simulink model "oloop2"  (Simulink 3.00)
settings: Solver=ode45  SolverMode=SingleTasking  StartTime=0.0  StopTime=60  MaxStep=1  RelTol=1e-7  AbsTol=1e-7
undefined symbols (not defined in the file): sfunyst, uaero0, uprop0
libraries: fbuttons x5, fdclib10 x1, wndlib2 x1
settings Model: SaveTime=off  SaveOutput=off  RTWTemplateMakefile=grt_vc.tmf  LastModifiedBy=Dutchroll

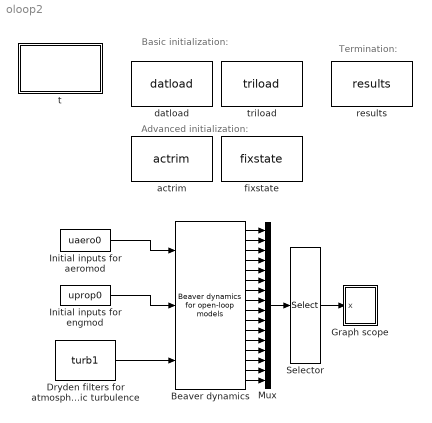
== system oloop2 ==
  note: Basic initialization:
  note: Termination:
  note: Advanced initialization:
  Beaver dynamics : fdclib10/Beaver dynamics  for open-loop models
  Dryden filters for atmospheric turbulence : wndlib2/turb1
  Graph scope : Subsystem  mask(Storage scope.){npts=100, color='g-'}
      mask prompts: npts "Initial Time Range:"; color "Initial y-min:"
      mask help:
      | Storage scope using MATLAB graph window.
      | Enter plotting ranges and line type.
      mask init:
      | close all; ax = [0, @1, @2, @3];
      mask Help: Uses MATLAB's graph window.\nUse only one block per system.\nLine type must be in quotes.\nSee the M-file sfunyst.m.
      mask Display: plot(0,0,100,100,[83,76,63,52,42,38,28,16,11,84,11,11,11,90,90,11],[75,58,47,54,72,80,84,74,65,65,65,90,40,40,90,90])
  Initial inputs for aeromod : Constant  Value=uaero0
  Initial inputs for engmod : Constant  Value=uprop0
  Mux : Mux  Inputs=16
  Selector : Selector  Elements=8  InputPortWidth=16
  actrim : fbuttons/actrim
  datload : fbuttons/datload
  fixstate : fbuttons/fixstate
  results : fbuttons/results
  t : Subsystem
      settings: OpenFcn=browse oloop
      mask Display: disp('OLOOP2\nMarc Rauw\nMay 2003')
  triload : fbuttons/triload
  wires:
  Dryden filters for atmospheric turbulence/1 -> Beaver dynamics/3
  Initial inputs for engmod/1 -> Beaver dynamics/2
  Initial inputs for aeromod/1 -> Beaver dynamics/1
  Selector/1 -> Graph scope/1(x)
  Beaver dynamics/1 -> Mux/1
  Beaver dynamics/2 -> Mux/2
  Beaver dynamics/3 -> Mux/3
  Beaver dynamics/4 -> Mux/4
  Beaver dynamics/5 -> Mux/5
  Beaver dynamics/6 -> Mux/6
  Beaver dynamics/7 -> Mux/7
  Beaver dynamics/8 -> Mux/8
  Beaver dynamics/9 -> Mux/9
  Beaver dynamics/10 -> Mux/10
  Beaver dynamics/11 -> Mux/11
  Beaver dynamics/12 -> Mux/12
  Beaver dynamics/13 -> Mux/13
  Beaver dynamics/14 -> Mux/14
  Beaver dynamics/15 -> Mux/15
  Beaver dynamics/16 -> Mux/16
  Mux/1 -> Selector/1

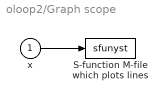
== system oloop2/Graph scope ==
  x : Inport  Port=1  PortWidth=-1  SampleTime=-1  DataType=auto
      settings: SignalType=auto
  "S-function M-file which plots lines " : S-Function  LoadFcn=sfunyst([],[],[],'LoadBlock')  FunctionName=sfunyst  Parameters=ax, color, npts  PortCounts=[]  SFunctionModules=''
      settings: CopyFcn=sfunyst([],[],[],'CopyBlock')  DeleteFcn=sfunyst([],[],[],'DeleteBlock')
  wires:
  x/1 -> "S-function M-file which plots lines "/1

== system oloop2/t ==
